simulink model "trygit"  (R2020b)
settings: Solver=VariableStepAuto  StartTime=0.0  StopTime=10.0  RelTol=1e-3
settings Model: Creator=GURU  LastModifiedBy=GURU

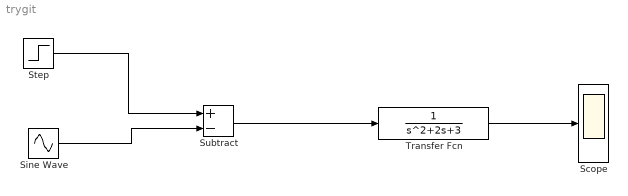
== system trygit ==
  Scope : Scope
  Sine Wave : Sin  SampleTime=0
  Step : Step  SampleTime=0
  Subtract : Sum  Inputs=+-
  Transfer Fcn : TransferFcn  Denominator=[1 2 3]
  wires:
  Step/1 -> Subtract/1
  Sine Wave/1 -> Subtract/2
  Subtract/1 -> Transfer Fcn/1
  Transfer Fcn/1 -> Scope/1
